simulink library "FilterLib"  (R2012b)
settings: Solver=ode45  StartTime=0.0  StopTime=10.0  RelTol=1e-3
undefined symbols (not defined in the file): bw, Fs, N
libraries: dspsigops x1
settings Model: Creator=klindqvi  LastModifiedBy=klindqvi

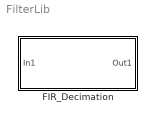
== system FilterLib ==
  FIR_Decimation : Subsystem  TreatAsAtomicUnit=on  RTWFcnName=FIR_Decimation  mask{coefficients=fir1(N, (bw/(Fs/2))*[1 2])}
      mask prompts: coefficients "filter coefficients"
      settings: RTWFcnNameOpts=User specified

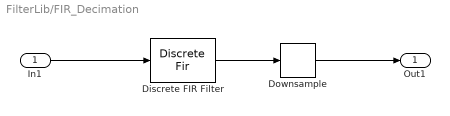
== system FilterLib/FIR_Decimation ==
  In1 : Inport
  Discrete FIR Filter : DiscreteFir  Coefficients=coefficients
  Downsample : dspsigops/Downsample  N=89  phase=0  InputProcessing=Columns as channels (frame based)  RateOptions=Allow multirate processing  smode=Allow multirate  fmode=Maintain input frame size  ic=0
  Out1 : Outport
  wires:
  In1/1 -> Discrete FIR Filter/1
  Downsample/1 -> Out1/1
  Discrete FIR Filter/1 -> Downsample/1
